simulink model "BME_project_EMK"  (R2020a)
settings: Solver=VariableStepAuto  StartTime=0.0  StopTime=20  RelTol=1e-3
settings Model: Creator=sunda  LastModifiedBy=sunda

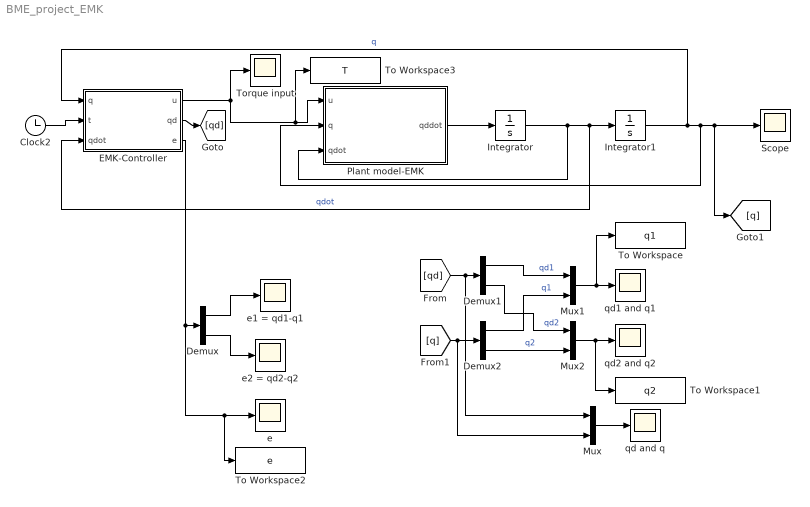
== system BME_project_EMK ==
  Clock2 : Clock
  Demux : Demux  Outputs=2
  Demux1 : Demux  Outputs=2
  Demux2 : Demux  Outputs=2
  EMK-Controller : MATLAB Function  TreatAsAtomicUnit=on
  Integrator : Integrator  InitialCondition=zeros(2,1)
  Integrator1 : Integrator  InitialCondition=zeros(2,1)
  Mux : Mux  Inputs=2
  Mux1 : Mux  Inputs=2
  Mux2 : Mux  Inputs=2
  Plant model-EMK : MATLAB Function  TreatAsAtomicUnit=on
  Scope : Scope
  To Workspace : ToWorkspace  VariableName=q1  SaveFormat=Timeseries  SampleTime=-1
  To Workspace1 : ToWorkspace  VariableName=q2  SaveFormat=Timeseries  SampleTime=-1
  To Workspace2 : ToWorkspace  VariableName=e  SaveFormat=Timeseries  SampleTime=-1
  To Workspace3 : ToWorkspace  VariableName=T  SaveFormat=Timeseries  SampleTime=-1
  Torque input : Scope
  e : Scope
  e1 = qd1-q1 : Scope
  e2 = qd2-q2 : Scope
  qd and q : Scope
  qd1 and q1 : Scope
  qd2 and q2 : Scope
  wires:
  Plant model-EMK/1(qddot) -> Integrator/1
  Integrator/1 -> Plant model-EMK/3(qdot), Integrator1/1, EMK-Controller/3(qdot)  "qdot"
  Integrator1/1 -> EMK-Controller/1(q), [q], Scope/1, Plant model-EMK/2(q)  "q"
  Clock2/1 -> EMK-Controller/2(t)
  EMK-Controller/1(u) -> Torque input/1, To Workspace3/1, Plant model-EMK/1(u)
  EMK-Controller/3(e) -> To Workspace2/1, e/1, Demux/1
  Mux1/1 -> To Workspace/1, qd1 and q1/1
  Demux/1 -> e1 = qd1-q1/1
  Demux/2 -> e2 = qd2-q2/1
  EMK-Controller/2(qd) -> [qd]
  [qd] -> Mux/1, Demux1/1
  [q] -> Mux/2, Demux2/1
  Demux1/1 -> Mux1/1  "qd1"
  Demux2/1 -> Mux1/2  "q1"
  Demux1/2 -> Mux2/1  "qd2"
  Mux2/1 -> To Workspace1/1, qd2 and q2/1
  Demux2/2 -> Mux2/2  "q2"
  Mux/1 -> qd and q/1

== matlab function BME_project_EMK/EMK-Controller ==
  data: q input; u output; t input; qdot input; qd output; e output
%% Exact model knowledge controller

function [u,qd,e] = fcn(q,t,qdot)

q1 = q(1);
q2 = q(2);

q1dot =qdot(1);
q2dot = qdot(2);

p1 = 3.473; %%% kg.m^2
p2 = 0.196; %%% kg.m^2
p3 = 0.242; %%% kg.m^2

fd1 = 5.3; %%% N.m.sec
fd2 = 1.1; %%% N.m.sec

%%% Inertia matrix M(q)
M =[p1+2*p3*cos(q2)     p2 + p3*cos(q2);...
    p2 + p3* cos(q2)        p2];

%%% Centripetal and Coriollis term V(q,qdot)

Vm = [-p3*sin(q2)*q2dot     -p3*sin(q2)*(q1dot +q2dot);...
     p3* sin(q2)*q1dot                  0];
 
%%% Damping/ friction term 

Fd = [fd1   0;
      0     fd2];
  
qd = [cos(t) cos(2*t)]';
qd_dot = [-sin(t) -2*sin(2*t)]';
qd_ddot = [-cos(t) -4*cos(2*t)]';

e = qd-q;
e_dot =qd_dot - qdot;


% Gain values

alpha = 5; 
K = 5*eye(2);

r = e_dot + alpha*e;
 
%%% Control law - EMK

u = M*qd_ddot + Vm*qdot+alpha*M*e_dot+Fd*qdot+Vm*r+K*r;

end

== matlab function BME_project_EMK/Plant model-EMK ==
  data: u input; q input; qdot input; qddot output
%% Robot Plant model - EMK
function qddot = fcn(u,q,qdot)

q1 = q(1);
q2 = q(2);

q1dot =qdot(1);
q2dot = qdot(2);

p1 = 3.473; %%% kg.m^2
p2 = 0.196; %%% kg.m^2
p3 = 0.242; %%% kg.m^2

fd1 = 5.3; %%% N.m.sec
fd2 = 1.1; %%% N.m.sec

Td1 = 0;   %%% N.m
Td2 = 0;   %%% N.m
%%% Inertia matrix M(q)
M =[p1+2*p3*cos(q2)     p2 + p3*cos(q2);...
    p2 + p3* cos(q2)        p2];

%%% Centripetal and Coriollis term V(q,qdot)

Vm = [-p3*sin(q2)*q2dot     -p3*sin(q2)*(q1dot +q2dot);...
     p3* sin(q2)*q1dot                  0];
 
%%% Damping/ friction term 

Fd = [fd1   0;
      0     fd2];
  
%%% Disturbance:

Td = [Td1 Td2]';
%%% Robot dynamics of a Two - link Robot

qddot = inv(M)*(u - Vm*qdot -Fd*qdot - Td);

end
